simulink subsystem "controller_subsystem"  (R2024b)
settings: Solver=VariableStepAuto  StartTime=0.0  StopTime=10.0  RelTol=1e-3
undefined symbols (not defined in the file or in its folder): samplingrate
settings Model: Creator=finnb  LastModifiedBy=finnb

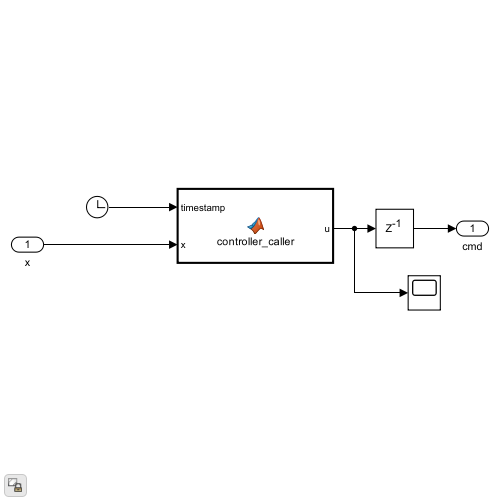
[thumbnail: Simulink's stored preview of the top-level diagram]
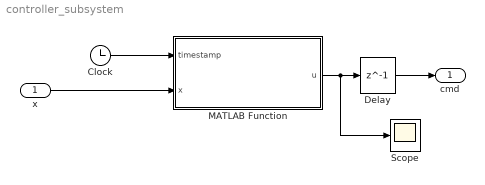
== system controller_subsystem ==
  x : Inport
  Clock : Clock
  Delay : Delay  DelayLength=1  InputProcessing=Columns as channels (frame based)  SampleTime=samplingrate
  MATLAB Function : MATLAB Function  TreatAsAtomicUnit=on
  Scope : Scope
  cmd : Outport
  wires:
  x/1 -> MATLAB Function/2(x)
  Clock/1 -> MATLAB Function/1(timestamp)
  MATLAB Function/1(u) -> Delay/1, Scope/1
  Delay/1 -> cmd/1

== matlab function controller_subsystem/MATLAB Function ==
  settings: updateMethod=DISCRETE  sampleTime=samplingrate
  data: timestamp input; x input; u output
function u = controller_caller(timestamp, x)
    u = 0;
    u = controller_module(timestamp, x);
end
